simulink subsystem "Controllers"  (R2024b)
settings: Solver=VariableStepAuto  StartTime=0.0  StopTime=10.0  RelTol=1e-3
undefined symbols (not defined in the file): CarrierFreq, dend, DiscIntNeverNeededParam, freq_left, freq_right, Ll, nb_cell, numberOfCell, numd, P_AC, Rl, Tctrl, Ts, V_AC_sec
libraries: powerlib_extras x12, simulink x12
(part 4 of 4)

== matlab function Controllers/pulsegen_VBC1/VBC/VBC3/MATLAB Function ==
  data: gate_in input; go output; int output; Vc input; ichg input; Nref input; errV input; g_his input; inti input; nbc input
function [go,int]= fcn(gate_in,Vc,ichg,Nref,errV,g_his,inti, nbc)

go =gate_in;

NbON =sum(gate_in );


int =[0 ; 0 ];


if NbON >=nbc
    go =ones(size(gate_in));
elseif NbON <=0
    go =zeros (size (gate_in ));
else
    if(inti (1 )>=1 )&&(inti (1 )<=nbc )
        g_his (inti (1 ))=inti (2 );
    end
    if length(g_his) ~= nbc
        gg =gate_in ;

    else
        gg =g_his ;
    end
    NbON_his =sum (g_his );
    event =NbON -NbON_his ;
    aloop0 =1 ;
    aloop1 =1 ;
    idx_m0 =1 ; idx_m1 =1 ;
    for ii =[1 :nbc ]
        if(event >=0 ) && (gg(ii) < 0.5 )
            if(aloop0 ==1 )
                if event >1
                    gg(ii )=1 ;
                    event =event -1 ;
                else
                    idx_m0 =ii ;
                    aloop0 =0 ;
                end
            else

                if (ichg >0 )==(Vc(ii )<Vc (idx_m0 ))
                    idx_m0 =ii ;
                end
            end
        elseif (event<=0 )&&(gg(ii )>0.5 )
            if(aloop1 ==1 )
                if event <-1
                    gg(ii )=0 ;
                    event =event +1 ;
                else
                    idx_m1 =ii ;
                    aloop1 =0 ;
                end
            else


                if (ichg >0 )~=(Vc (ii )<Vc (idx_m1 ))
                    idx_m1 =ii ;
                end
            end
        else

        end
    end
    if (event >0 )
        gg (idx_m0 )=event ;
        if event <1
            int (1 )=idx_m0 ;
            int (2 )=1 ;
        end
    elseif (event < 0)
        gg (idx_m1 )=1 +event ;
        if event >-1
            int (1 )=idx_m1 ;
            int (2 )=0 ;
        end
    else
        if(ichg >0 )
            Vdel =-Vc(idx_m0 ) + Vc(idx_m1 );
        else
            Vdel =Vc(idx_m0 ) - Vc(idx_m1 );
        end
        if (Vdel /(Vc(idx_m0 ) + Vc(idx_m1 ))>errV )
            gg (idx_m0 )=1 ;
            gg (idx_m1 )=0 ;
        end
    end
    go =gg ;
end

== matlab function Controllers/pulsegen_VBC1/VBC/VBC4/MATLAB Function ==
  data: gate_in input; go output; int output; Vc input; ichg input; Nref input; errV input; g_his input; inti input; nbc input
function [go,int]= fcn(gate_in,Vc,ichg,Nref,errV,g_his,inti, nbc)

go =gate_in;

NbON =sum(gate_in );


int =[0 ; 0 ];


if NbON >=nbc
    go =ones(size(gate_in));
elseif NbON <=0
    go =zeros (size (gate_in ));
else
    if(inti (1 )>=1 )&&(inti (1 )<=nbc )
        g_his (inti (1 ))=inti (2 );
    end
    if length(g_his) ~= nbc
        gg =gate_in ;

    else
        gg =g_his ;
    end
    NbON_his =sum (g_his );
    event =NbON -NbON_his ;
    aloop0 =1 ;
    aloop1 =1 ;
    idx_m0 =1 ; idx_m1 =1 ;
    for ii =[1 :nbc ]
        if(event >=0 ) && (gg(ii) < 0.5 )
            if(aloop0 ==1 )
                if event >1
                    gg(ii )=1 ;
                    event =event -1 ;
                else
                    idx_m0 =ii ;
                    aloop0 =0 ;
                end
            else

                if (ichg >0 )==(Vc(ii )<Vc (idx_m0 ))
                    idx_m0 =ii ;
                end
            end
        elseif (event<=0 )&&(gg(ii )>0.5 )
            if(aloop1 ==1 )
                if event <-1
                    gg(ii )=0 ;
                    event =event +1 ;
                else
                    idx_m1 =ii ;
                    aloop1 =0 ;
                end
            else


                if (ichg >0 )~=(Vc (ii )<Vc (idx_m1 ))
                    idx_m1 =ii ;
                end
            end
        else

        end
    end
    if (event >0 )
        gg (idx_m0 )=event ;
        if event <1
            int (1 )=idx_m0 ;
            int (2 )=1 ;
        end
    elseif (event < 0)
        gg (idx_m1 )=1 +event ;
        if event >-1
            int (1 )=idx_m1 ;
            int (2 )=0 ;
        end
    else
        if(ichg >0 )
            Vdel =-Vc(idx_m0 ) + Vc(idx_m1 );
        else
            Vdel =Vc(idx_m0 ) - Vc(idx_m1 );
        end
        if (Vdel /(Vc(idx_m0 ) + Vc(idx_m1 ))>errV )
            gg (idx_m0 )=1 ;
            gg (idx_m1 )=0 ;
        end
    end
    go =gg ;
end

== matlab function Controllers/pulsegen_VBC1/VBC/VBC2/MATLAB Function ==
  data: gate_in input; go output; int output; Vc input; ichg input; Nref input; errV input; g_his input; inti input; nbc input
function [go,int]= fcn(gate_in,Vc,ichg,Nref,errV,g_his,inti, nbc)

go =gate_in;

NbON =sum(gate_in );


int =[0 ; 0 ];


if NbON >=nbc
    go =ones(size(gate_in));
elseif NbON <=0
    go =zeros (size (gate_in ));
else
    if(inti (1 )>=1 )&&(inti (1 )<=nbc )
        g_his (inti (1 ))=inti (2 );
    end
    if length(g_his) ~= nbc
        gg =gate_in ;

    else
        gg =g_his ;
    end
    NbON_his =sum (g_his );
    event =NbON -NbON_his ;
    aloop0 =1 ;
    aloop1 =1 ;
    idx_m0 =1 ; idx_m1 =1 ;
    for ii =[1 :nbc ]
        if(event >=0 ) && (gg(ii) < 0.5 )
            if(aloop0 ==1 )
                if event >1
                    gg(ii )=1 ;
                    event =event -1 ;
                else
                    idx_m0 =ii ;
                    aloop0 =0 ;
                end
            else

                if (ichg >0 )==(Vc(ii )<Vc (idx_m0 ))
                    idx_m0 =ii ;
                end
            end
        elseif (event<=0 )&&(gg(ii )>0.5 )
            if(aloop1 ==1 )
                if event <-1
                    gg(ii )=0 ;
                    event =event +1 ;
                else
                    idx_m1 =ii ;
                    aloop1 =0 ;
                end
            else


                if (ichg >0 )~=(Vc (ii )<Vc (idx_m1 ))
                    idx_m1 =ii ;
                end
            end
        else

        end
    end
    if (event >0 )
        gg (idx_m0 )=event ;
        if event <1
            int (1 )=idx_m0 ;
            int (2 )=1 ;
        end
    elseif (event < 0)
        gg (idx_m1 )=1 +event ;
        if event >-1
            int (1 )=idx_m1 ;
            int (2 )=0 ;
        end
    else
        if(ichg >0 )
            Vdel =-Vc(idx_m0 ) + Vc(idx_m1 );
        else
            Vdel =Vc(idx_m0 ) - Vc(idx_m1 );
        end
        if (Vdel /(Vc(idx_m0 ) + Vc(idx_m1 ))>errV )
            gg (idx_m0 )=1 ;
            gg (idx_m1 )=0 ;
        end
    end
    go =gg ;
end

== matlab function Controllers/pulsegen_VBC1/VBC/VBC5/MATLAB Function ==
  data: gate_in input; go output; int output; Vc input; ichg input; Nref input; errV input; g_his input; inti input; nbc input
function [go,int]= fcn(gate_in,Vc,ichg,Nref,errV,g_his,inti, nbc)

go =gate_in;

NbON =sum(gate_in );


int =[0 ; 0 ];


if NbON >=nbc
    go =ones(size(gate_in));
elseif NbON <=0
    go =zeros (size (gate_in ));
else
    if(inti (1 )>=1 )&&(inti (1 )<=nbc )
        g_his (inti (1 ))=inti (2 );
    end
    if length(g_his) ~= nbc
        gg =gate_in ;

    else
        gg =g_his ;
    end
    NbON_his =sum (g_his );
    event =NbON -NbON_his ;
    aloop0 =1 ;
    aloop1 =1 ;
    idx_m0 =1 ; idx_m1 =1 ;
    for ii =[1 :nbc ]
        if(event >=0 ) && (gg(ii) < 0.5 )
            if(aloop0 ==1 )
                if event >1
                    gg(ii )=1 ;
                    event =event -1 ;
                else
                    idx_m0 =ii ;
                    aloop0 =0 ;
                end
            else

                if (ichg >0 )==(Vc(ii )<Vc (idx_m0 ))
                    idx_m0 =ii ;
                end
            end
        elseif (event<=0 )&&(gg(ii )>0.5 )
            if(aloop1 ==1 )
                if event <-1
                    gg(ii )=0 ;
                    event =event +1 ;
                else
                    idx_m1 =ii ;
                    aloop1 =0 ;
                end
            else


                if (ichg >0 )~=(Vc (ii )<Vc (idx_m1 ))
                    idx_m1 =ii ;
                end
            end
        else

        end
    end
    if (event >0 )
        gg (idx_m0 )=event ;
        if event <1
            int (1 )=idx_m0 ;
            int (2 )=1 ;
        end
    elseif (event < 0)
        gg (idx_m1 )=1 +event ;
        if event >-1
            int (1 )=idx_m1 ;
            int (2 )=0 ;
        end
    else
        if(ichg >0 )
            Vdel =-Vc(idx_m0 ) + Vc(idx_m1 );
        else
            Vdel =Vc(idx_m0 ) - Vc(idx_m1 );
        end
        if (Vdel /(Vc(idx_m0 ) + Vc(idx_m1 ))>errV )
            gg (idx_m0 )=1 ;
            gg (idx_m1 )=0 ;
        end
    end
    go =gg ;
end

== matlab function Controllers/pulsegen_VBC1/VBC/VBC6/MATLAB Function ==
  data: gate_in input; go output; int output; Vc input; ichg input; Nref input; errV input; g_his input; inti input; nbc input
function [go,int]= fcn(gate_in,Vc,ichg,Nref,errV,g_his,inti, nbc)

go =gate_in;

NbON =sum(gate_in );


int =[0 ; 0 ];


if NbON >=nbc
    go =ones(size(gate_in));
elseif NbON <=0
    go =zeros (size (gate_in ));
else
    if(inti (1 )>=1 )&&(inti (1 )<=nbc )
        g_his (inti (1 ))=inti (2 );
    end
    if length(g_his) ~= nbc
        gg =gate_in ;

    else
        gg =g_his ;
    end
    NbON_his =sum (g_his );
    event =NbON -NbON_his ;
    aloop0 =1 ;
    aloop1 =1 ;
    idx_m0 =1 ; idx_m1 =1 ;
    for ii =[1 :nbc ]
        if(event >=0 ) && (gg(ii) < 0.5 )
            if(aloop0 ==1 )
                if event >1
                    gg(ii )=1 ;
                    event =event -1 ;
                else
                    idx_m0 =ii ;
                    aloop0 =0 ;
                end
            else

                if (ichg >0 )==(Vc(ii )<Vc (idx_m0 ))
                    idx_m0 =ii ;
                end
            end
        elseif (event<=0 )&&(gg(ii )>0.5 )
            if(aloop1 ==1 )
                if event <-1
                    gg(ii )=0 ;
                    event =event +1 ;
                else
                    idx_m1 =ii ;
                    aloop1 =0 ;
                end
            else


                if (ichg >0 )~=(Vc (ii )<Vc (idx_m1 ))
                    idx_m1 =ii ;
                end
            end
        else

        end
    end
    if (event >0 )
        gg (idx_m0 )=event ;
        if event <1
            int (1 )=idx_m0 ;
            int (2 )=1 ;
        end
    elseif (event < 0)
        gg (idx_m1 )=1 +event ;
        if event >-1
            int (1 )=idx_m1 ;
            int (2 )=0 ;
        end
    else
        if(ichg >0 )
            Vdel =-Vc(idx_m0 ) + Vc(idx_m1 );
        else
            Vdel =Vc(idx_m0 ) - Vc(idx_m1 );
        end
        if (Vdel /(Vc(idx_m0 ) + Vc(idx_m1 ))>errV )
            gg (idx_m0 )=1 ;
            gg (idx_m1 )=0 ;
        end
    end
    go =gg ;
end

== matlab function Controllers/sorting Tmuxed/MATLAB Function VBC1 case 8 ==
  data: in input; ind output
function ind   = fcn(in)
%#codegen

[out, ind] = sort(in)

== matlab function Controllers/pulsegen_VBC2/VBC/VBC1/MATLAB Function ==
  data: gate_in input; go output; int output; Vc input; ichg input; Nref input; errV input; g_his input; inti input; nbc input
function [go,int]= fcn(gate_in,Vc,ichg,Nref,errV,g_his,inti, nbc)

go =gate_in;

NbON =sum(gate_in );


int =[0 ; 0 ];


if NbON >=nbc
    go =ones(size(gate_in));
elseif NbON <=0
    go =zeros (size (gate_in ));
else
    if(inti (1 )>=1 )&&(inti (1 )<=nbc )
        g_his (inti (1 ))=inti (2 );
    end
    if length(g_his) ~= nbc
        gg =gate_in ;

    else
        gg =g_his ;
    end
    NbON_his =sum (g_his );
    event =NbON -NbON_his ;
    aloop0 =1 ;
    aloop1 =1 ;
    idx_m0 =1 ; idx_m1 =1 ;
    for ii =[1 :nbc ]
        if(event >=0 ) && (gg(ii) < 0.5 )
            if(aloop0 ==1 )
                if event >1
                    gg(ii )=1 ;
                    event =event -1 ;
                else
                    idx_m0 =ii ;
                    aloop0 =0 ;
                end
            else

                if (ichg >0 )==(Vc(ii )<Vc (idx_m0 ))
                    idx_m0 =ii ;
                end
            end
        elseif (event<=0 )&&(gg(ii )>0.5 )
            if(aloop1 ==1 )
                if event <-1
                    gg(ii )=0 ;
                    event =event +1 ;
                else
                    idx_m1 =ii ;
                    aloop1 =0 ;
                end
            else


                if (ichg >0 )~=(Vc (ii )<Vc (idx_m1 ))
                    idx_m1 =ii ;
                end
            end
        else

        end
    end
    if (event >0 )
        gg (idx_m0 )=event ;
        if event <1
            int (1 )=idx_m0 ;
            int (2 )=1 ;
        end
    elseif (event < 0)
        gg (idx_m1 )=1 +event ;
        if event >-1
            int (1 )=idx_m1 ;
            int (2 )=0 ;
        end
    else
        if(ichg >0 )
            Vdel =-Vc(idx_m0 ) + Vc(idx_m1 );
        else
            Vdel =Vc(idx_m0 ) - Vc(idx_m1 );
        end
        if (Vdel /(Vc(idx_m0 ) + Vc(idx_m1 ))>errV )
            gg (idx_m0 )=1 ;
            gg (idx_m1 )=0 ;
        end
    end
    go =gg ;
end

== matlab function Controllers/pulsegen_VBC2/VBC/VBC2/MATLAB Function ==
  data: gate_in input; go output; int output; Vc input; ichg input; Nref input; errV input; g_his input; inti input; nbc input
function [go,int]= fcn(gate_in,Vc,ichg,Nref,errV,g_his,inti, nbc)

go =gate_in;

NbON =sum(gate_in );


int =[0 ; 0 ];


if NbON >=nbc
    go =ones(size(gate_in));
elseif NbON <=0
    go =zeros (size (gate_in ));
else
    if(inti (1 )>=1 )&&(inti (1 )<=nbc )
        g_his (inti (1 ))=inti (2 );
    end
    if length(g_his) ~= nbc
        gg =gate_in ;

    else
        gg =g_his ;
    end
    NbON_his =sum (g_his );
    event =NbON -NbON_his ;
    aloop0 =1 ;
    aloop1 =1 ;
    idx_m0 =1 ; idx_m1 =1 ;
    for ii =[1 :nbc ]
        if(event >=0 ) && (gg(ii) < 0.5 )
            if(aloop0 ==1 )
                if event >1
                    gg(ii )=1 ;
                    event =event -1 ;
                else
                    idx_m0 =ii ;
                    aloop0 =0 ;
                end
            else

                if (ichg >0 )==(Vc(ii )<Vc (idx_m0 ))
                    idx_m0 =ii ;
                end
            end
        elseif (event<=0 )&&(gg(ii )>0.5 )
            if(aloop1 ==1 )
                if event <-1
                    gg(ii )=0 ;
                    event =event +1 ;
                else
                    idx_m1 =ii ;
                    aloop1 =0 ;
                end
            else


                if (ichg >0 )~=(Vc (ii )<Vc (idx_m1 ))
                    idx_m1 =ii ;
                end
            end
        else

        end
    end
    if (event >0 )
        gg (idx_m0 )=event ;
        if event <1
            int (1 )=idx_m0 ;
            int (2 )=1 ;
        end
    elseif (event < 0)
        gg (idx_m1 )=1 +event ;
        if event >-1
            int (1 )=idx_m1 ;
            int (2 )=0 ;
        end
    else
        if(ichg >0 )
            Vdel =-Vc(idx_m0 ) + Vc(idx_m1 );
        else
            Vdel =Vc(idx_m0 ) - Vc(idx_m1 );
        end
        if (Vdel /(Vc(idx_m0 ) + Vc(idx_m1 ))>errV )
            gg (idx_m0 )=1 ;
            gg (idx_m1 )=0 ;
        end
    end
    go =gg ;
end

== matlab function Controllers/pulsegen_VBC2/VBC/VBC3/MATLAB Function ==
  data: gate_in input; go output; int output; Vc input; ichg input; Nref input; errV input; g_his input; inti input; nbc input
function [go,int]= fcn(gate_in,Vc,ichg,Nref,errV,g_his,inti, nbc)

go =gate_in;

NbON =sum(gate_in );


int =[0 ; 0 ];


if NbON >=nbc
    go =ones(size(gate_in));
elseif NbON <=0
    go =zeros (size (gate_in ));
else
    if(inti (1 )>=1 )&&(inti (1 )<=nbc )
        g_his (inti (1 ))=inti (2 );
    end
    if length(g_his) ~= nbc
        gg =gate_in ;

    else
        gg =g_his ;
    end
    NbON_his =sum (g_his );
    event =NbON -NbON_his ;
    aloop0 =1 ;
    aloop1 =1 ;
    idx_m0 =1 ; idx_m1 =1 ;
    for ii =[1 :nbc ]
        if(event >=0 ) && (gg(ii) < 0.5 )
            if(aloop0 ==1 )
                if event >1
                    gg(ii )=1 ;
                    event =event -1 ;
                else
                    idx_m0 =ii ;
                    aloop0 =0 ;
                end
            else

                if (ichg >0 )==(Vc(ii )<Vc (idx_m0 ))
                    idx_m0 =ii ;
                end
            end
        elseif (event<=0 )&&(gg(ii )>0.5 )
            if(aloop1 ==1 )
                if event <-1
                    gg(ii )=0 ;
                    event =event +1 ;
                else
                    idx_m1 =ii ;
                    aloop1 =0 ;
                end
            else


                if (ichg >0 )~=(Vc (ii )<Vc (idx_m1 ))
                    idx_m1 =ii ;
                end
            end
        else

        end
    end
    if (event >0 )
        gg (idx_m0 )=event ;
        if event <1
            int (1 )=idx_m0 ;
            int (2 )=1 ;
        end
    elseif (event < 0)
        gg (idx_m1 )=1 +event ;
        if event >-1
            int (1 )=idx_m1 ;
            int (2 )=0 ;
        end
    else
        if(ichg >0 )
            Vdel =-Vc(idx_m0 ) + Vc(idx_m1 );
        else
            Vdel =Vc(idx_m0 ) - Vc(idx_m1 );
        end
        if (Vdel /(Vc(idx_m0 ) + Vc(idx_m1 ))>errV )
            gg (idx_m0 )=1 ;
            gg (idx_m1 )=0 ;
        end
    end
    go =gg ;
end

== matlab function Controllers/pulsegen_VBC2/VBC/VBC4/MATLAB Function ==
  data: gate_in input; go output; int output; Vc input; ichg input; Nref input; errV input; g_his input; inti input; nbc input
function [go,int]= fcn(gate_in,Vc,ichg,Nref,errV,g_his,inti, nbc)

go =gate_in;

NbON =sum(gate_in );


int =[0 ; 0 ];


if NbON >=nbc
    go =ones(size(gate_in));
elseif NbON <=0
    go =zeros (size (gate_in ));
else
    if(inti (1 )>=1 )&&(inti (1 )<=nbc )
        g_his (inti (1 ))=inti (2 );
    end
    if length(g_his) ~= nbc
        gg =gate_in ;

    else
        gg =g_his ;
    end
    NbON_his =sum (g_his );
    event =NbON -NbON_his ;
    aloop0 =1 ;
    aloop1 =1 ;
    idx_m0 =1 ; idx_m1 =1 ;
    for ii =[1 :nbc ]
        if(event >=0 ) && (gg(ii) < 0.5 )
            if(aloop0 ==1 )
                if event >1
                    gg(ii )=1 ;
                    event =event -1 ;
                else
                    idx_m0 =ii ;
                    aloop0 =0 ;
                end
            else

                if (ichg >0 )==(Vc(ii )<Vc (idx_m0 ))
                    idx_m0 =ii ;
                end
            end
        elseif (event<=0 )&&(gg(ii )>0.5 )
            if(aloop1 ==1 )
                if event <-1
                    gg(ii )=0 ;
                    event =event +1 ;
                else
                    idx_m1 =ii ;
                    aloop1 =0 ;
                end
            else


                if (ichg >0 )~=(Vc (ii )<Vc (idx_m1 ))
                    idx_m1 =ii ;
                end
            end
        else

        end
    end
    if (event >0 )
        gg (idx_m0 )=event ;
        if event <1
            int (1 )=idx_m0 ;
            int (2 )=1 ;
        end
    elseif (event < 0)
        gg (idx_m1 )=1 +event ;
        if event >-1
            int (1 )=idx_m1 ;
            int (2 )=0 ;
        end
    else
        if(ichg >0 )
            Vdel =-Vc(idx_m0 ) + Vc(idx_m1 );
        else
            Vdel =Vc(idx_m0 ) - Vc(idx_m1 );
        end
        if (Vdel /(Vc(idx_m0 ) + Vc(idx_m1 ))>errV )
            gg (idx_m0 )=1 ;
            gg (idx_m1 )=0 ;
        end
    end
    go =gg ;
end

== matlab function Controllers/pulsegen_VBC2/VBC/VBC5/MATLAB Function ==
  data: gate_in input; go output; int output; Vc input; ichg input; Nref input; errV input; g_his input; inti input; nbc input
function [go,int]= fcn(gate_in,Vc,ichg,Nref,errV,g_his,inti, nbc)

go =gate_in;

NbON =sum(gate_in );


int =[0 ; 0 ];


if NbON >=nbc
    go =ones(size(gate_in));
elseif NbON <=0
    go =zeros (size (gate_in ));
else
    if(inti (1 )>=1 )&&(inti (1 )<=nbc )
        g_his (inti (1 ))=inti (2 );
    end
    if length(g_his) ~= nbc
        gg =gate_in ;

    else
        gg =g_his ;
    end
    NbON_his =sum (g_his );
    event =NbON -NbON_his ;
    aloop0 =1 ;
    aloop1 =1 ;
    idx_m0 =1 ; idx_m1 =1 ;
    for ii =[1 :nbc ]
        if(event >=0 ) && (gg(ii) < 0.5 )
            if(aloop0 ==1 )
                if event >1
                    gg(ii )=1 ;
                    event =event -1 ;
                else
                    idx_m0 =ii ;
                    aloop0 =0 ;
                end
            else

                if (ichg >0 )==(Vc(ii )<Vc (idx_m0 ))
                    idx_m0 =ii ;
                end
            end
        elseif (event<=0 )&&(gg(ii )>0.5 )
            if(aloop1 ==1 )
                if event <-1
                    gg(ii )=0 ;
                    event =event +1 ;
                else
                    idx_m1 =ii ;
                    aloop1 =0 ;
                end
            else


                if (ichg >0 )~=(Vc (ii )<Vc (idx_m1 ))
                    idx_m1 =ii ;
                end
            end
        else

        end
    end
    if (event >0 )
        gg (idx_m0 )=event ;
        if event <1
            int (1 )=idx_m0 ;
            int (2 )=1 ;
        end
    elseif (event < 0)
        gg (idx_m1 )=1 +event ;
        if event >-1
            int (1 )=idx_m1 ;
            int (2 )=0 ;
        end
    else
        if(ichg >0 )
            Vdel =-Vc(idx_m0 ) + Vc(idx_m1 );
        else
            Vdel =Vc(idx_m0 ) - Vc(idx_m1 );
        end
        if (Vdel /(Vc(idx_m0 ) + Vc(idx_m1 ))>errV )
            gg (idx_m0 )=1 ;
            gg (idx_m1 )=0 ;
        end
    end
    go =gg ;
end

== matlab function Controllers/pulsegen_VBC2/VBC/VBC6/MATLAB Function ==
  data: gate_in input; go output; int output; Vc input; ichg input; Nref input; errV input; g_his input; inti input; nbc input
function [go,int]= fcn(gate_in,Vc,ichg,Nref,errV,g_his,inti, nbc)

go =gate_in;

NbON =sum(gate_in );


int =[0 ; 0 ];


if NbON >=nbc
    go =ones(size(gate_in));
elseif NbON <=0
    go =zeros (size (gate_in ));
else
    if(inti (1 )>=1 )&&(inti (1 )<=nbc )
        g_his (inti (1 ))=inti (2 );
    end
    if length(g_his) ~= nbc
        gg =gate_in ;

    else
        gg =g_his ;
    end
    NbON_his =sum (g_his );
    event =NbON -NbON_his ;
    aloop0 =1 ;
    aloop1 =1 ;
    idx_m0 =1 ; idx_m1 =1 ;
    for ii =[1 :nbc ]
        if(event >=0 ) && (gg(ii) < 0.5 )
            if(aloop0 ==1 )
                if event >1
                    gg(ii )=1 ;
                    event =event -1 ;
                else
                    idx_m0 =ii ;
                    aloop0 =0 ;
                end
            else

                if (ichg >0 )==(Vc(ii )<Vc (idx_m0 ))
                    idx_m0 =ii ;
                end
            end
        elseif (event<=0 )&&(gg(ii )>0.5 )
            if(aloop1 ==1 )
                if event <-1
                    gg(ii )=0 ;
                    event =event +1 ;
                else
                    idx_m1 =ii ;
                    aloop1 =0 ;
                end
            else


                if (ichg >0 )~=(Vc (ii )<Vc (idx_m1 ))
                    idx_m1 =ii ;
                end
            end
        else

        end
    end
    if (event >0 )
        gg (idx_m0 )=event ;
        if event <1
            int (1 )=idx_m0 ;
            int (2 )=1 ;
        end
    elseif (event < 0)
        gg (idx_m1 )=1 +event ;
        if event >-1
            int (1 )=idx_m1 ;
            int (2 )=0 ;
        end
    else
        if(ichg >0 )
            Vdel =-Vc(idx_m0 ) + Vc(idx_m1 );
        else
            Vdel =Vc(idx_m0 ) - Vc(idx_m1 );
        end
        if (Vdel /(Vc(idx_m0 ) + Vc(idx_m1 ))>errV )
            gg (idx_m0 )=1 ;
            gg (idx_m1 )=0 ;
        end
    end
    go =gg ;
end

== matlab function Controllers/pulsegen_VBC1/VBC/VBC1/MATLAB Function ==
  data: gate_in input; go output; int output; Vc input; ichg input; Nref input; errV input; g_his input; inti input; nbc input
function [go,int]= fcn(gate_in,Vc,ichg,Nref,errV,g_his,inti, nbc)

go =gate_in;

NbON =sum(gate_in );


int =[0 ; 0 ];


if NbON >=nbc
    go =ones(size(gate_in));
elseif NbON <=0
    go =zeros (size (gate_in ));
else
    if(inti (1 )>=1 )&&(inti (1 )<=nbc )
        g_his (inti (1 ))=inti (2 );
    end
    if length(g_his) ~= nbc
        gg =gate_in ;

    else
        gg =g_his ;
    end
    NbON_his =sum (g_his );
    event =NbON -NbON_his ;
    aloop0 =1 ;
    aloop1 =1 ;
    idx_m0 =1 ; idx_m1 =1 ;
    for ii =[1 :nbc ]
        if(event >=0 ) && (gg(ii) < 0.5 )
            if(aloop0 ==1 )
                if event >1
                    gg(ii )=1 ;
                    event =event -1 ;
                else
                    idx_m0 =ii ;
                    aloop0 =0 ;
                end
            else

                if (ichg >0 )==(Vc(ii )<Vc (idx_m0 ))
                    idx_m0 =ii ;
                end
            end
        elseif (event<=0 )&&(gg(ii )>0.5 )
            if(aloop1 ==1 )
                if event <-1
                    gg(ii )=0 ;
                    event =event +1 ;
                else
                    idx_m1 =ii ;
                    aloop1 =0 ;
                end
            else


                if (ichg >0 )~=(Vc (ii )<Vc (idx_m1 ))
                    idx_m1 =ii ;
                end
            end
        else

        end
    end
    if (event >0 )
        gg (idx_m0 )=event ;
        if event <1
            int (1 )=idx_m0 ;
            int (2 )=1 ;
        end
    elseif (event < 0)
        gg (idx_m1 )=1 +event ;
        if event >-1
            int (1 )=idx_m1 ;
            int (2 )=0 ;
        end
    else
        if(ichg >0 )
            Vdel =-Vc(idx_m0 ) + Vc(idx_m1 );
        else
            Vdel =Vc(idx_m0 ) - Vc(idx_m1 );
        end
        if (Vdel /(Vc(idx_m0 ) + Vc(idx_m1 ))>errV )
            gg (idx_m0 )=1 ;
            gg (idx_m1 )=0 ;
        end
    end
    go =gg ;
end
